simulink model "bai1"  (R2015a)
settings: Solver=ode45  StartTime=0.0  StopTime=10.0  FixedStep=1e-5  RelTol=1e-3
libraries: dsparch4 x1
settings Model: Creator=Win 10  LastModifiedBy=Win 10

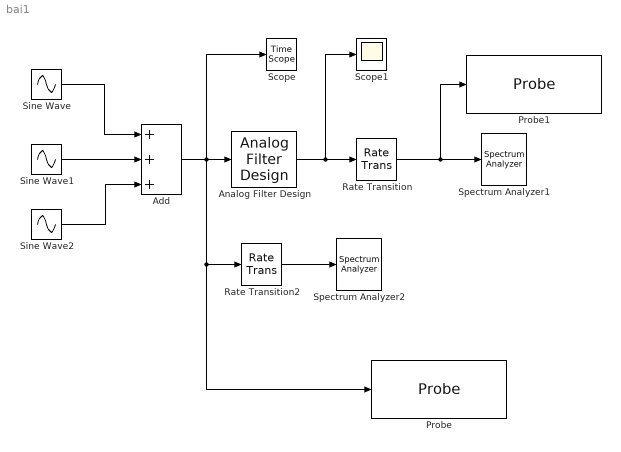
== system bai1 ==
  Add : Sum  Inputs=+++
  Analog Filter Design : dsparch4/Analog Filter Design  method=Butterworth  filttype=Lowpass  N=9  Wlo=1000  Whi=80  Rp=2  Rs=40
  Probe : Probe  ProbeWidth=off  ProbeComplexSignal=off  ProbeSignalDimensions=on
  Probe1 : Probe  ProbeWidth=off  ProbeComplexSignal=off  ProbeSignalDimensions=on
  Rate Transition : RateTransition  Deterministic=off  OutPortSampleTime=1/262144
  Rate Transition2 : RateTransition  Deterministic=off  OutPortSampleTime=1/262144
  Scope : TimeScope
  Scope1 : Scope
      settings: TimeRange=0.01227706298828757  YMin=-2  YMax=2
  Sine Wave : Sin  Amplitude=2  Frequency=500  SampleTime=1e-5  VectorParams1D=off
  Sine Wave1 : Sin  Frequency=1500  SampleTime=1e-5  VectorParams1D=off
  Sine Wave2 : Sin  Amplitude=0.5  Frequency=2500  SampleTime=1e-5  VectorParams1D=off
  Spectrum Analyzer1 : SpectrumAnalyzer
  Spectrum Analyzer2 : SpectrumAnalyzer
  wires:
  Sine Wave/1 -> Add/1
  Sine Wave1/1 -> Add/2
  Sine Wave2/1 -> Add/3
  Analog Filter Design/1 -> Scope1/1, Rate Transition/1
  Rate Transition/1 -> Spectrum Analyzer1/1, Probe1/1
  Add/1 -> Probe/1, Rate Transition2/1, Analog Filter Design/1, Scope/1
  Rate Transition2/1 -> Spectrum Analyzer2/1
